simulink model "ReatorChernobylControlado"  (R2025b)
settings: Solver=VariableStepAuto  StartTime=0.0  StopTime=10.0  RelTol=1e-3
values from neighbouring files (symbols this model uses):
  beta = calculaBeta(planta)    [avaliaLGR.m]    (also in avaliaNyquist.m; avaliarReatorChernobyl.m; avaliarReatorChernobylComControlador.m = planta.beta_total; avaliarReatorChernobylControlado.m)
  denC = 1    [avaliarReatorChernobylControlado.m]
  numC = K    [avaliarReatorChernobylControlado.m]
  planta = obterPlantaReatorNuclear    [avaliaLGR.m]    (also in avaliaNyquist.m; avaliarReatorChernobyl.m; avaliarReatorChernobylComControlador.m = obterPlantaReator; avaliarReatorChernobylControlado.m = SimulaFalhaChernobyl(planta))
undefined symbols (not defined in the file or in its folder): denG0, denGm, denGtheta, denGv, numG0, numGm, numGtheta, numGv
settings Model: Creator=danilo  LastModifiedBy=danilo

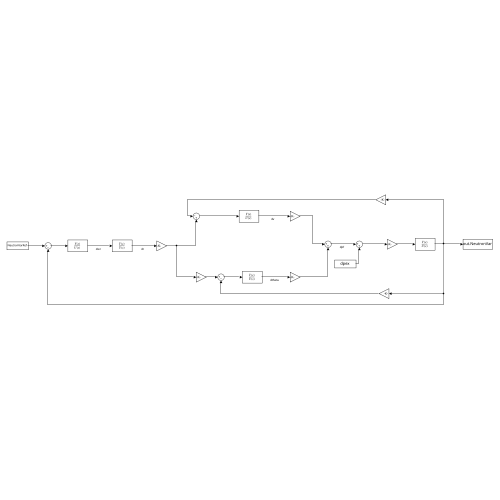
[thumbnail: Simulink's stored preview of the top-level diagram]
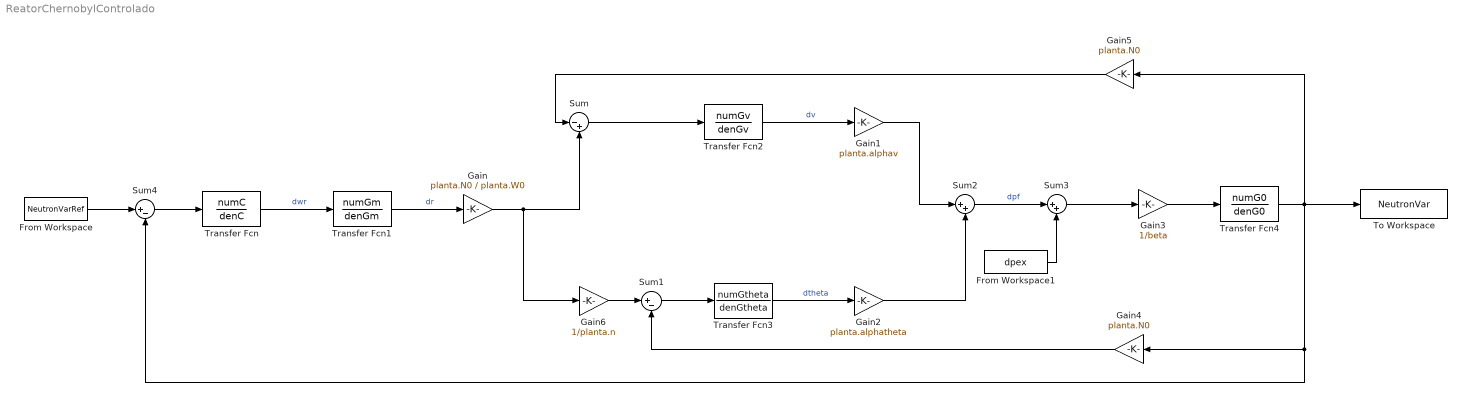
== system ReatorChernobylControlado ==
  From Workspace : FromWorkspace  VariableName=NeutronVarRef
  From Workspace1 : FromWorkspace  VariableName=dpex
  Gain : Gain  Gain=planta.N0 / planta.W0
  Gain1 : Gain  Gain=planta.alphav
  Gain2 : Gain  Gain=planta.alphatheta
  Gain3 : Gain  Gain=1/beta
  Gain4 : Gain  Gain=planta.N0
  Gain5 : Gain  Gain=planta.N0
  Gain6 : Gain  Gain=1/planta.n
  Sum : Sum  Inputs=|-+
  Sum1 : Sum  Inputs=|+-
  Sum2 : Sum  Inputs=|++
  Sum3 : Sum  Inputs=|++
  Sum4 : Sum  Inputs=|+-
  To Workspace : ToWorkspace  VariableName=NeutronVar  SaveFormat=Timeseries  SampleTime=-1
  Transfer Fcn : TransferFcn  Numerator=numC  Denominator=denC
  Transfer Fcn1 : TransferFcn  Numerator=numGm  Denominator=denGm
  Transfer Fcn2 : TransferFcn  Numerator=numGv  Denominator=denGv
  Transfer Fcn3 : TransferFcn  Numerator=numGtheta  Denominator=denGtheta
  Transfer Fcn4 : TransferFcn  Numerator=numG0  Denominator=denG0
  wires:
  Gain6/1 -> Sum1/1
  From Workspace/1 -> Sum4/1
  Sum4/1 -> Transfer Fcn/1
  Transfer Fcn/1 -> Transfer Fcn1/1  "dwr"
  Transfer Fcn1/1 -> Gain/1  "dr"
  Gain/1 -> Gain6/1, Sum/2
  Sum1/1 -> Transfer Fcn3/1
  Transfer Fcn3/1 -> Gain2/1  "dtheta"
  Sum/1 -> Transfer Fcn2/1
  Transfer Fcn2/1 -> Gain1/1  "dv"
  Gain1/1 -> Sum2/1
  Gain2/1 -> Sum2/2
  Sum2/1 -> Sum3/1  "dpf"
  Sum3/1 -> Gain3/1
  Gain3/1 -> Transfer Fcn4/1
  Transfer Fcn4/1 -> Sum4/2, Gain4/1, Gain5/1, To Workspace/1
  Gain5/1 -> Sum/1
  Gain4/1 -> Sum1/2
  From Workspace1/1 -> Sum3/2
